simulink model "WK3_Problem1"  (R2023a)
settings: Solver=FixedStepAuto  StartTime=0.0  StopTime=10.0  FixedStep=0.01  RelTol=1e-3
values from neighbouring files (symbols this model uses):
  a1 = 2    [NathanielMalmontWK3Lab.m]
  b1 = 3    [NathanielMalmontWK3Lab.m]
  c1 = 0.25    [NathanielMalmontWK3Lab.m]
  d1 = 1*rad    (= 6.283185)    [NathanielMalmontWK3Lab.m]
settings Model: Creator=natha  LastModifiedBy=natha

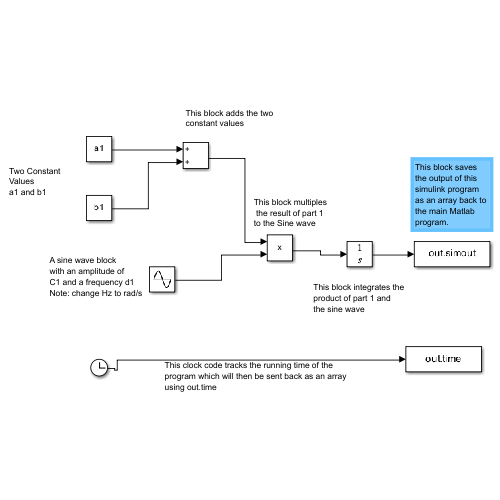
[thumbnail: Simulink's stored preview of the top-level diagram]
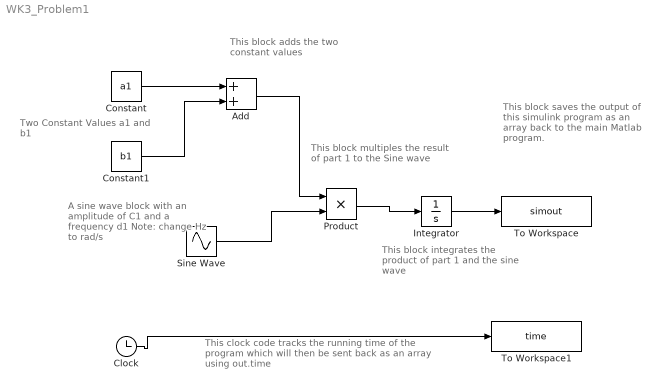
== system WK3_Problem1 ==
  note: This clock code tracks the running time of the
      | program which will then be sent back as an array
      | using out.time
  note: This block saves
      | the output of this
      | simulink program
      | as an array back to
      | the main Matlab
      | program.
  note: This block integrates the
      | product of part 1 and
      | the sine wave
  note: This block multiples
      |  the result of part 1
      | to the Sine wave
  note: A sine wave block
      | with an amplitude of
      | C1 and a frequency d1
      | Note: change Hz to rad/s
  note: This block adds the two
      | constant values
  note: Two Constant
      | Values
      | a1 and b1
  Add : Sum
  Clock : Clock
  Constant : Constant  Value=a1
  Constant1 : Constant  Value=b1
  Integrator : Integrator
  Product : Product
  Sine Wave : Sin  Amplitude=c1  Frequency=d1  SampleTime=0
  To Workspace : ToWorkspace  VariableName=simout  SampleTime=-1
  To Workspace1 : ToWorkspace  VariableName=time  SampleTime=-1
  wires:
  Constant/1 -> Add/1
  Constant1/1 -> Add/2
  Add/1 -> Product/1
  Sine Wave/1 -> Product/2
  Product/1 -> Integrator/1
  Integrator/1 -> To Workspace/1
  Clock/1 -> To Workspace1/1
